simulink model "HexaMotor_System_Identification_V02"  (R2026a)
settings: Solver=FixedStepDiscrete  StopTime=5.0904  FixedStep=0.005  EnableMultiTasking=on
undefined symbols (not defined in the file or in its folder): sampleRate
libraries: arduinolib x3, arduinosensorlib x1, eeGeneralControl x1, simulink x1
settings Model: SimulationMode=external  SILPILModeSetting=veronly  ExtModeTrigDuration=2  Creator=bkhusain  LastModifiedBy=arkad
settings OptimizationCC: PassReuseOutputArgsThreshold=0.0
settings DebuggingCC: ParameterOverflowMsg=none  ParameterUnderflowMsg=error  ParameterPrecisionLossMsg=none
settings HardwareCC: ProdLargestAtomicInteger=Long  ProdLargestAtomicFloat=Double  ProdHWDeviceType=ARM Compatible->ARM Cortex
settings RTWCC: SystemTargetFile=ert.tlc  HardwareBoard=Arduino MKRZero  TLCOptions=-aInlineSetEventsForThisBaseRateFcn=TLC_FALSE -aSuppressMultiTaskScheduler=TLC_FALSE -aRateBasedStepFcn=1  Toolchain=Arduino ARM  BuildConfiguration=Faster Runs  Description=Embedded Coder
settings ERTTargetCC: ExtModeTransport=3.0  ExtModeAutomaticAllocSize=off  ExtModeStaticAllocSize=8192.0  DynamicArrayContainerType=coder::array  ERTCustomFileBanners=off  SupportContinuousTime=on  SupportNonInlinedSFcns=on  SupportVariableSizeSignals=on  ModelStepFunctionPrototypeControlCompliant=off
settings SimscapeCC: SimscapeNominalValues="[{\"value\":\"1\",\"unit\":\"A\"},{\"value\":\"1\",\"unit\":\"bar\"},{\"value\":\"1\",\"unit\":\"cm^2\"},{\"value\":\"1\",\"unit\":\"cm^3/s\"},{\"value\":\"1\",\"unit\":\"kJ/kg\"},{\"value\":\"1\",\"unit\":\"kW\"},{\"value\":\"1\",\"unit\":\"l\"},{\"value\":\"1\",\"unit\":\"N\"},{\"value\":\"1\",\"unit\":\"N*m\"},{\"value\":\"1\",\"unit\":\"V\"}]"  SimscapeLogType=none  SimscapeLogDataHistory=5000.0

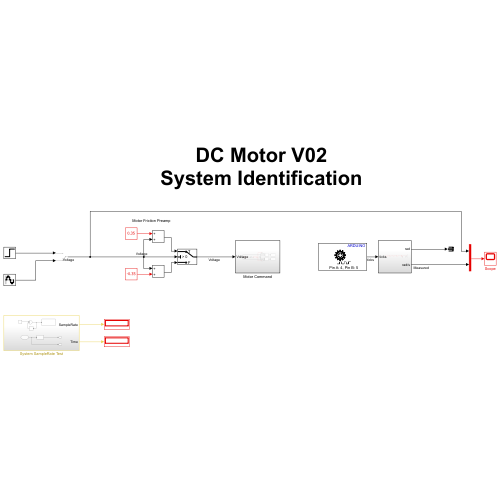
[thumbnail: Simulink's stored preview of the top-level diagram]
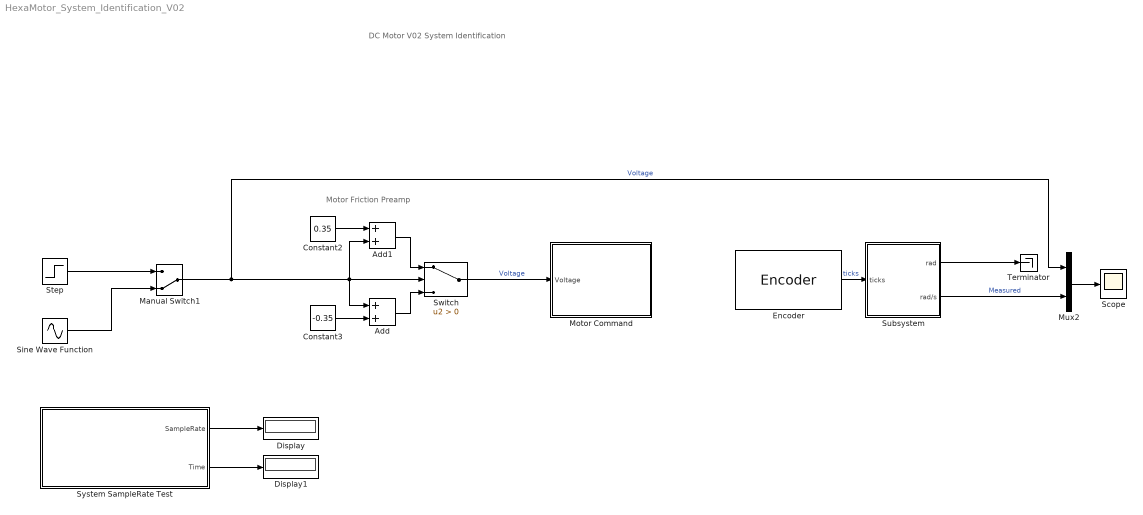
== system HexaMotor_System_Identification_V02 ==
  note: DC Motor V02
      | System Identification
  note: Motor Friction Preamp
  Add : Sum
  Add1 : Sum
  Constant2 : Constant  Value=0.35  SampleTime=-1
  Constant3 : Constant  Value=-0.35  SampleTime=-1
  Display : Display
  Display1 : Display
  Encoder : arduinosensorlib/Encoder  InputA=4  InputB=5  Mode=No reset  SampleTime=-1
  Manual Switch1 : ManualSwitch  CurrentSetting=0
  Motor Command : Subsystem
  Mux2 : Mux  Inputs=2
  Scope : Scope
      settings: TimeSpan=5.0904  ActiveDisplayYMinimum=-3.1703117441656365  ActiveDisplayYMaximum=21.18805406353675
  Sine Wave Function : Sin  Amplitude=7  Frequency=7  SampleTime=sampleRate
  Step : Step  FinalValue=7  SampleTime=sampleRate
  Subsystem : Subsystem
  Switch : Switch  Criteria=u2 > Threshold  SaturateOnIntegerOverflow=off  InputSameDT=off
  System SampleRate Test : Subsystem
  Terminator : Terminator
  wires:
  System SampleRate Test/1(SampleRate) -> Display/1
  System SampleRate Test/2(Time) -> Display1/1
  Mux2/1 -> Scope/1
  Step/1 -> Manual Switch1/1
  Sine Wave Function/1 -> Manual Switch1/2
  Manual Switch1/1 -> Mux2/1, Add1/2, Switch/2, Add/1  "Voltage"
  Add/1 -> Switch/3
  Switch/1 -> Motor Command/1(Voltage)  "Voltage"
  Constant2/1 -> Add1/1
  Constant3/1 -> Add/2
  Add1/1 -> Switch/1
  Encoder/1 -> Subsystem/1(ticks)  "ticks"
  Subsystem/1(rad) -> Terminator/1
  Subsystem/2(rad/s) -> Mux2/2  "Measured"

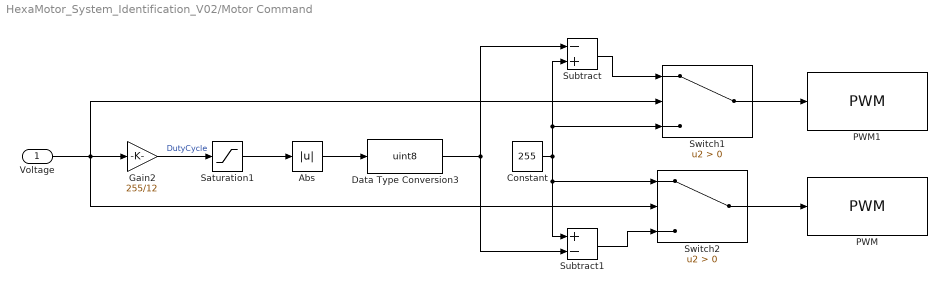
== system HexaMotor_System_Identification_V02/Motor Command ==
  Voltage : Inport
  Abs : Abs  SaturateOnIntegerOverflow=off
  Constant : Constant  Value=255  OutDataTypeStr=uint8  SampleTime=-1
  Data Type Conversion3 : DataTypeConversion  OutDataTypeStr=uint8  SaturateOnIntegerOverflow=off  RndMeth=Floor
  Gain2 : Gain  Gain=255/12
  PWM : arduinolib/PWM  pinNumber=2  frequencyType=Specify  desiredFrequency=5000  achievableFrequency=5000
      settings: LibrarySourceBlock=gizmoLibrary/Arduino Utilities/PWM
  PWM1 : arduinolib/PWM  pinNumber=3  frequencyType=Specify  desiredFrequency=5000  achievableFrequency=5000
      settings: LibrarySourceBlock=gizmoLibrary/Arduino Utilities/PWM
  Saturation1 : Saturate  UpperLimit=255  LowerLimit=-255
  Subtract : Sum  Inputs=-+
  Subtract1 : Sum  Inputs=+-
  Switch1 : Switch  Criteria=u2 > Threshold  OutDataTypeStr=uint8  SaturateOnIntegerOverflow=off  InputSameDT=off
  Switch2 : Switch  Criteria=u2 > Threshold  OutDataTypeStr=uint8  SaturateOnIntegerOverflow=off  InputSameDT=off
  wires:
  Voltage/1 -> Switch2/2, Switch1/2, Gain2/1
  Abs/1 -> Data Type Conversion3/1
  Subtract/1 -> Switch1/1
  Gain2/1 -> Saturation1/1  "DutyCycle"
  Subtract1/1 -> Switch2/3
  Constant/1 -> Switch1/3, Subtract/2, Subtract1/1, Switch2/1
  Data Type Conversion3/1 -> Subtract/1, Subtract1/2
  Saturation1/1 -> Abs/1
  Switch1/1 -> PWM1/1
  Switch2/1 -> PWM/1

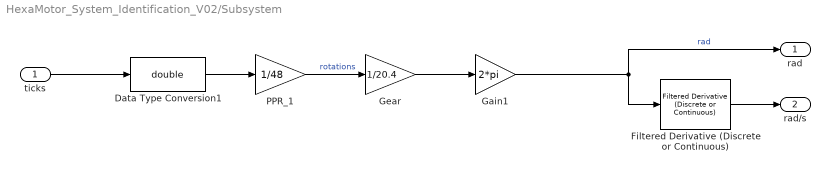
== system HexaMotor_System_Identification_V02/Subsystem ==
  ticks : Inport
  Data Type Conversion1 : DataTypeConversion  OutDataTypeStr=double  SaturateOnIntegerOverflow=off  RndMeth=Floor
  Filtered Derivative (Discrete or Continuous) : eeGeneralControl/Filtered Derivative (Discrete or Continuous)  K=1  T=0.05  B=inf  A=-inf  minRatio=10  init_option=Inherited from block input  x0=0  Ts=-1
      settings: LibrarySourceBlock=|
      | ee_sl_lib/General Control/Filtered Derivative
      | (Discrete or Continuous)
  Gain1 : Gain  Gain=2*pi
  Gear : Gain  Gain=1/20.4
  PPR_1 : Gain  Gain=1/48
  rad : Outport
  rad/s : Outport  Port=2
  wires:
  PPR_1/1 -> Gear/1  "rotations"
  Data Type Conversion1/1 -> PPR_1/1
  ticks/1 -> Data Type Conversion1/1
  Gear/1 -> Gain1/1
  Gain1/1 -> rad/1, Filtered Derivative (Discrete or Continuous)/1  "rad"
  Filtered Derivative (Discrete or Continuous)/1 -> rad/s/1

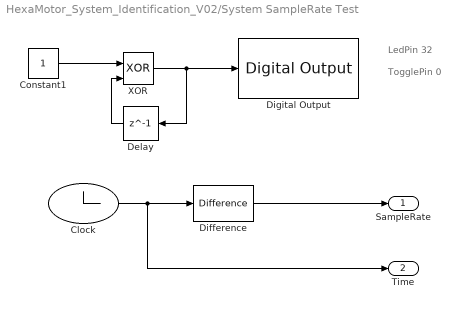
== system HexaMotor_System_Identification_V02/System SampleRate Test ==
  note: LedPin 32
  note: TogglePin 0
  Clock : Clock
      settings: Decimation=3
  Constant1 : Constant  SampleTime=-1
  Delay : Delay  DelayLength=1  InitialCondition=0
  Difference : simulink/Quick Insert/Discrete/Difference  ICPrevInput=0.0  OutMin=[]  OutMax=[]  OutDataType=fixdt(1, 16)  OutScaling=2^-10  DoSatur=off
  Digital Output : arduinolib/Digital Output  pinNumber=32  Direction=output  blockPlatform=arduino
  XOR : Logic  Operator=XOR  IconShape=distinctive  AllPortsSameDT=off  OutDataTypeStr=boolean
  SampleRate : Outport
  Time : Outport  Port=2
  wires:
  XOR/1 -> Delay/1, Digital Output/1
  Constant1/1 -> XOR/1
  Delay/1 -> XOR/2
  Clock/1 -> Time/1, Difference/1
  Difference/1 -> SampleRate/1
